simulink model "stabilnost_dc_motora"  (R2017b)
settings: Solver=VariableStepAuto  StartTime=0.0  StopTime=10.0  RelTol=1e-3
values from neighbouring files (symbols this model uses):
  Kp = 0.5    [a.m]
  Ti = 0.15    [a.m]
settings Model: Creator=USER  LastModifiedBy=USER

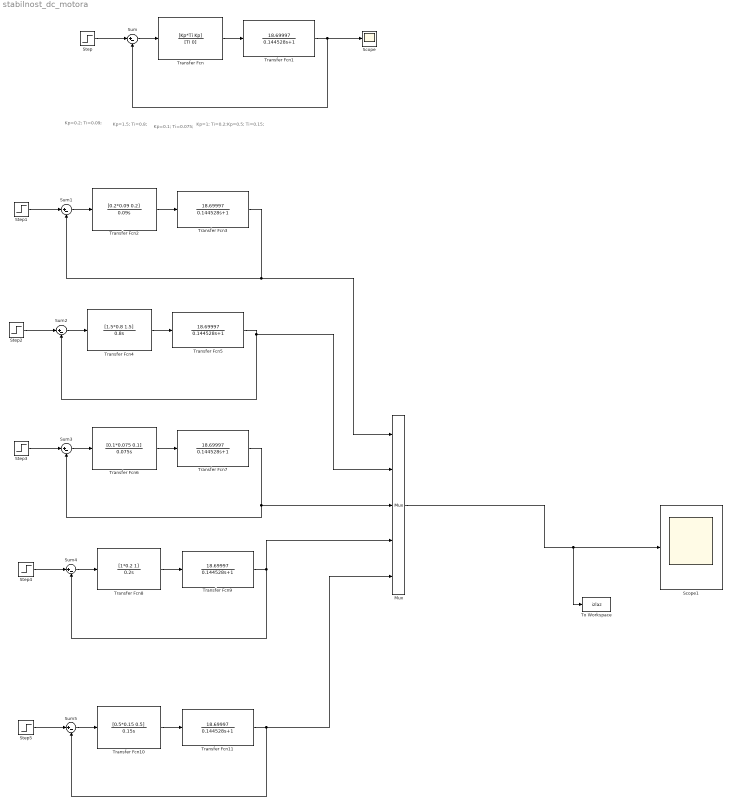
== system stabilnost_dc_motora ==
  note: Kp=0.2;
      | Ti=0.09;
  note: Kp=1.5;
      | Ti=0.8;
  note: Kp=0.1;
      | Ti=0.075;
  note: Kp=1;
      | Ti=0.2;
  note: Kp=0.5;
      | Ti=0.15;
  Mux : Mux  Inputs=5
  Scope : Scope
  Scope1 : Scope
  Step{,1..5} (6 alike) : Step  Time=0  SampleTime=0
  Sum{,1..5} (6 alike) : Sum  Inputs=|+-
  To Workspace : ToWorkspace  VariableName=izlaz  SampleTime=-1
  Transfer Fcn : TransferFcn  Numerator=[Kp*Ti Kp]  Denominator=[Ti 0]
  Transfer Fcn{1,3,5,7,9,11} (6 alike) : TransferFcn  Numerator=[18.69997]  Denominator=[0.144528 1]
  Transfer Fcn10 : TransferFcn  Numerator=[0.5*0.15 0.5]  Denominator=[0.15 0]
  Transfer Fcn2 : TransferFcn  Numerator=[0.2*0.09 0.2]  Denominator=[0.09 0]
  Transfer Fcn4 : TransferFcn  Numerator=[1.5*0.8 1.5]  Denominator=[0.8 0]
  Transfer Fcn6 : TransferFcn  Numerator=[0.1*0.075 0.1]  Denominator=[0.075 0]
  Transfer Fcn8 : TransferFcn  Numerator=[1*0.2 1]  Denominator=[0.2 0]
  wires:
  Transfer Fcn1/1 -> Sum/2, Scope/1
  Transfer Fcn/1 -> Transfer Fcn1/1
  Sum/1 -> Transfer Fcn/1
  Step/1 -> Sum/1
  Step1/1 -> Sum1/1
  Sum1/1 -> Transfer Fcn2/1
  Transfer Fcn2/1 -> Transfer Fcn3/1
  Transfer Fcn3/1 -> Mux/1, Sum1/2
  Transfer Fcn5/1 -> Mux/2, Sum2/2
  Transfer Fcn4/1 -> Transfer Fcn5/1
  Sum2/1 -> Transfer Fcn4/1
  Step2/1 -> Sum2/1
  Step3/1 -> Sum3/1
  Sum3/1 -> Transfer Fcn6/1
  Transfer Fcn6/1 -> Transfer Fcn7/1
  Transfer Fcn7/1 -> Mux/3, Sum3/2
  Transfer Fcn9/1 -> Mux/4, Sum4/2
  Transfer Fcn8/1 -> Transfer Fcn9/1
  Sum4/1 -> Transfer Fcn8/1
  Step4/1 -> Sum4/1
  Step5/1 -> Sum5/1
  Sum5/1 -> Transfer Fcn10/1
  Transfer Fcn10/1 -> Transfer Fcn11/1
  Transfer Fcn11/1 -> Mux/5, Sum5/2
  Mux/1 -> To Workspace/1, Scope1/1
